simulink model "rotacao"  (R2016a)
settings: Solver=ode4  SolverMode=SingleTasking  StartTime=0.0  StopTime=80  FixedStep=0.001  RelTol=1e-3
undefined symbols (not defined in the file or in its folder): DiscIntNeverNeededParam, sigbuilder_block
settings Model: SimulationMode=accelerator  Creator=colom  LastModifiedBy=ITA
settings SolverCC: AutoInsertRateTranBlk=on
settings DataIOCC: ReturnWorkspaceOutputs=on
settings DebuggingCC: UnconnectedInputMsg=none  UnconnectedOutputMsg=none  UnconnectedLineMsg=none  SFUnexpectedBacktrackingDiag=error  SFNoUnconditionalDefaultTransitionDiag=error
settings HardwareCC: ProdWordSize=32  ProdHWDeviceType=Specified
settings SFSimCC: SimUseLocalCustomCode=on
settings RTWCC: RTWUseLocalCustomCode=on
settings GRTTargetCC: TargetLangStandard=C99 (ISO)  GeneratePreprocessorConditionals=Use local settings
settings ConfigComp: CovMetricSettings=dwe  CovHtmlReporting=off  CovSaveCumulativeToWorkspaceVar=off  CovSaveSingleToWorkspaceVar=off  CovExternalEMLEnable=on

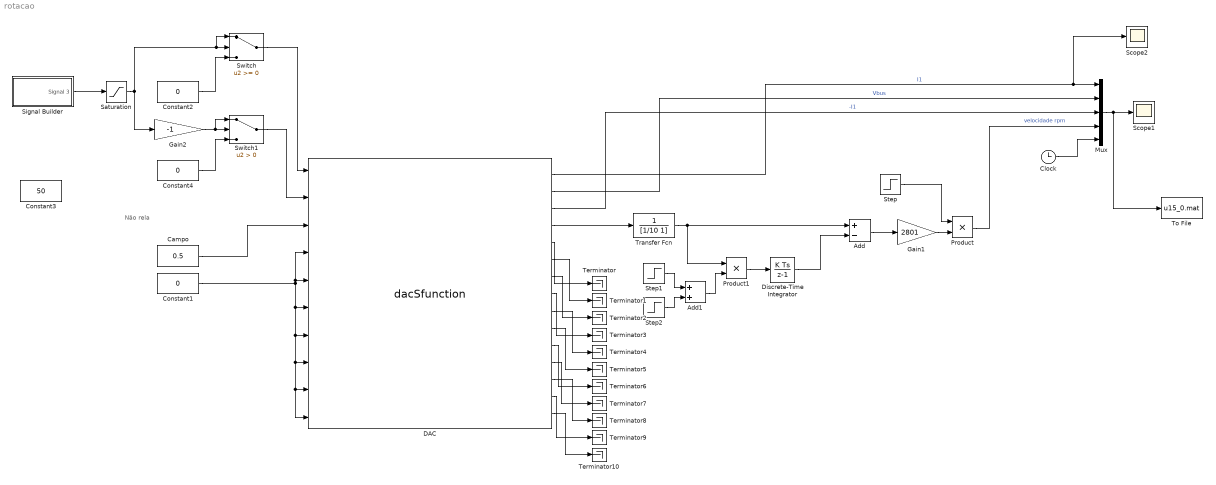
== system rotacao ==
  note: Não rela
  Add : Sum  Inputs=+-
  Add1 : Sum
  Campo : Constant  Value=0.5
  Clock : Clock
  Constant1 : Constant  Value=0
  Constant2 : Constant  Value=0
  Constant3 : Constant  Value=50
  Constant4 : Constant  Value=0
  DAC : S-Function  FunctionName=dacSfunction  Parameters=serialPort,sampleFreqHz,gpioCh1Mode,gpioCh1FinalState,gpioCh2Mode,gpioCh2FinalState,gpioCh3Mode,gpioCh3FinalState,gpioCh4Mode,gpioCh4FinalState,gpioCh5Mode,gpioCh5FinalState,gpioCh6Mode,gpioCh6FinalState,gpioCh7Mode,gpioCh7FinalState,pwmDeadTimeNs,pwmFrequencyHz,pwm1Mode,pwm1FastMode,pwm1ChPolarity,pwm1ChnPolarity,pwm1ChIdleState,pwm1ChnIdleState,pwm1FinalDuty,pwm2Mode,pwm2FastMode,pwm2ChPolarity,pwm2ChnPolarity,pwm2ChIdleState,pwm2ChnIdleState,pwm2FinalDuty,pwm3Mode,pwm3FastMode,pwm3ChPolarity,pwm3ChnPolarity,pwm3ChIdleState,pwm3ChnIdleState,pwm3FinalDuty,enc1Mode,enc1Quadrature,enc1Direction,enc1Filter,enc1ResetCount,enc2Mode,enc2Quadrature,enc2Direction,enc2Filter,enc2ResetCount,enc3Mode,enc3Quadrature,enc3Direction,enc3Filter,enc3ResetCount  SFunctionDeploymentMode=off  EnableBusSupport=off  mask{serialPort='COM4', sampleFreqHz=100, gpioCh1Mode=Input, gpioCh1FinalState=Low, gpioCh2Mode=Input, gpioCh2FinalState=Low, gpioCh3Mode=Output, gpioCh3FinalState=High, gpioCh4Mode=Input, gpioCh4FinalState=Low, gpioCh5Mode=Input, gpioCh5FinalState=Low, gpioCh6Mode=Input, gpioCh6FinalState=Low, gpioCh7Mode=Input, gpioCh7FinalState=Low, pwmFrequencyHz=20000, pwmDeadTimeNs=1000, pwm1Mode=Mode 1, pwm1FastMode=off, pwm1ChPolarity=HIGH, pwm1ChnPolarity=HIGH, pwm1ChIdleState=LOW, pwm1ChnIdleState=LOW, pwm1FinalDuty=0, pwm2Mode=Mode 1, pwm2FastMode=off, pwm2ChPolarity=HIGH, pwm2ChnPolarity=HIGH, pwm2ChIdleState=LOW, pwm2ChnIdleState=LOW, pwm2FinalDuty=0, pwm3Mode=Mode 1, pwm3FastMode=off, pwm3ChPolarity=HIGH, pwm3ChnPolarity=HIGH, pwm3ChIdleState=LOW, pwm3ChnIdleState=LOW, pwm3FinalDuty=0, enc1Mode=Counter, enc1Quadrature=High resolution, enc1Direction=Counter Clock Wise is positive, enc1Filter=15, enc1ResetCount=off, enc2Mode=Counter, enc2Quadrature=High resolution, enc2Direction=Counter Clock Wise is positive, enc2Filter=15, enc2ResetCount=off, enc3Mode=Counter, enc3Quadrature=High resolution, enc3Direction=Clock Wise is positive, enc3Filter=15, enc3ResetCount=off}
      mask prompts: serialPort "Serial port"; sampleFreqHz "Sample frequency (Hz)"; gpioCh1Mode "Mode"; gpioCh1FinalState "Final state"; gpioCh2Mode "Mode"; gpioCh2FinalState "Final state"; gpioCh3Mode "Mode"; gpioCh3FinalState "Final state"; gpioCh4Mode "Mode"; gpioCh4FinalState "Final state"; gpioCh5Mode "Mode"; gpioCh5FinalState "Final state"; gpioCh6Mode "Mode"; gpioCh6FinalState "Final state"; gpioCh7Mode "Mode"; gpioCh7FinalState "Final state"; pwmFrequencyHz "Frequency (Hz)"; pwmDeadTimeNs "Dead time (ns)"; pwm1Mode "Mode"; pwm1FastMode "Fast mode"; pwm1ChPolarity "CH polarity"; pwm1ChnPolarity "CHN polarity"; pwm1ChIdleState "CH idle state"; pwm1ChnIdleState "CHN idle state"; pwm1FinalDuty "Final duty"; pwm2Mode "Mode"; pwm2FastMode "Fast mode"; pwm2ChPolarity "CH polarity"; pwm2ChnPolarity "CHN polarity"; pwm2ChIdleState "CH idle state"; pwm2ChnIdleState "CHN idle state"; pwm2FinalDuty "Final duty"; pwm3Mode "Mode"; pwm3FastMode "Fast mode"; pwm3ChPolarity "CH polarity"; pwm3ChnPolarity "CHN polarity"; pwm3ChIdleState "CH idle state"; pwm3ChnIdleState "CHN idle state"; pwm3FinalDuty "Final duty"; enc1Mode "Mode"; enc1Quadrature "Resolution"; enc1Direction "Direction"; enc1Filter "Filter"; enc1ResetCount "Reset count"; enc2Mode "Mode"; enc2Quadrature "Resolution"; enc2Direction "Direction"; enc2Filter "Filter"; enc2ResetCount "Reset count"; enc3Mode "Mode"; enc3Quadrature "Resolution"; enc3Direction "Direction"; enc3Filter "Filter"; enc3ResetCount "Reset count"
      mask init:
      | % The first list item is initiated with 1 and not 0
      mask TypeOptions gpioCh1Mode: Input | Output
      mask TypeOptions gpioCh1FinalState: Low | High
      mask TypeOptions gpioCh2Mode: Input | Output
      mask TypeOptions gpioCh2FinalState: Low | High
      mask TypeOptions gpioCh3Mode: Input | Output
      mask TypeOptions gpioCh3FinalState: Low | High
      mask TypeOptions gpioCh4Mode: Input | Output
      mask TypeOptions gpioCh4FinalState: Low | High
      mask TypeOptions gpioCh5Mode: Input | Output
      mask TypeOptions gpioCh5FinalState: Low | High
      mask TypeOptions gpioCh6Mode: Input | Output
      mask TypeOptions gpioCh6FinalState: Low | High
      mask TypeOptions gpioCh7Mode: Input | Output
      mask TypeOptions gpioCh7FinalState: Low | High
      mask TypeOptions pwm1Mode: Mode 1 | Mode 2
      mask TypeOptions pwm1ChPolarity: LOW | HIGH
      mask TypeOptions pwm1ChnPolarity: LOW | HIGH
      mask TypeOptions pwm1ChIdleState: LOW | HIGH
      mask TypeOptions pwm1ChnIdleState: LOW | HIGH
      mask TypeOptions pwm2Mode: Mode 1 | Mode 2
      mask TypeOptions pwm2ChPolarity: LOW | HIGH
      mask TypeOptions pwm2ChnPolarity: LOW | HIGH
      mask TypeOptions pwm2ChIdleState: LOW | HIGH
      mask TypeOptions pwm2ChnIdleState: LOW | HIGH
      mask TypeOptions pwm3Mode: Mode 1 | Mode 2
      mask TypeOptions pwm3ChPolarity: LOW | HIGH
      mask TypeOptions pwm3ChnPolarity: LOW | HIGH
      mask TypeOptions pwm3ChIdleState: LOW | HIGH
      mask TypeOptions pwm3ChnIdleState: LOW | HIGH
      mask TypeOptions enc1Mode: Counter | Time measurement
      mask TypeOptions enc1Quadrature: Low resolution | High resolution
      mask TypeOptions enc1Direction: Counter Clock Wise is positive | Clock Wise is positive
      mask TypeOptions enc2Mode: Counter | Time measurement
      mask TypeOptions enc2Quadrature: Low resolution | High resolution
      mask TypeOptions enc2Direction: Counter Clock Wise is positive | Clock Wise is positive
      mask TypeOptions enc3Mode: Counter | Time measurement
      mask TypeOptions enc3Quadrature: Low resolution | High resolution
      mask TypeOptions enc3Direction: Counter Clock Wise is positive | Clock Wise is positive
      mask DialogControl DescTextVar Prompt: %<MaskDescription> OpenDAC configuration
      mask Display:
      | % Give names to the input ports
      | port_label('input',  1, 'PWM CH1 (PA8/PB13)');
      | port_label('input',  2, 'PWM CH2 (PA9/PB14)');
      | port_label('input',  3, 'PWM CH3 (PA10/PB15)');
      | port_label('input',  4, 'Digital Write CH1 (PC15)');
      | port_label('input',  5, 'Digital Write CH2 (PC14)');
      | port_label('input',  6, 'Digital Write CH3 (PC13)');
      | port_label('input',  7, 'Digital Write CH4 (PB9)');
      | port_label('input',  8, 'Digital Write CH5 (PB8)');
      | port_label('input',  9, 'Digital Write CH6 (PB1)');
      | port_label('input', 10, 'Digital Write CH7 (PB12)');
      | 
      | % Give names to the output ports
      | port_label('output',  1, 'Analog In CH1 (PA0)');
      | port_label('output',  2, 'Analog In CH2 (PA1)');
      | port_label('output',  3, 'Analog In CH3 (PA4)');
      | port_label('output',  4, 'Analog In CH4 (PB0)');
      | port_label('output',  5, 'Encoder 1 (PB6/PB7)');
      | port_label('output',  6, 'Encoder 2 (PA15/PB3)');
      | port_label('output',  7, 'Encoder 3 (PB4/PB5)');
      | port_label('output',  8, 'Digital Read CH1 (PC15)');
      | port_label('output',  9, 'Digital Read CH2 (PC14)');
      | port_label('output', 10, 'Digital Read CH3 (PC13)');
      | port_label('output', 11, 'Digital Read CH4 (PB9)');
      | port_label('output', 12, 'Digital Read CH5 (PB8)');
      | port_label('output', 13, 'Digital Read CH6 (PB1)');
      | port_label('output', 14, 'Digital Read CH7 (PB12)');
      | port_label('output', 15, 'Real Time Clock');
  Discrete-Time Integrator : DiscreteIntegrator  InitialConditionSetting=State (most efficient)  ICPrevOutput=DiscIntNeverNeededParam  ICPrevScaledInput=DiscIntNeverNeededParam
  Gain1 : Gain  Gain=2801
  Gain2 : Gain  Gain=-1
  Mux : Mux  Inputs=5
  Product : Product
  Product1 : Product
  Saturation : Saturate  UpperLimit=1  LowerLimit=-1
  Scope1 : Scope
  Scope2 : Scope
  Signal Builder : Subsystem  Tag=STV Subsys  LoadFcn=sigbuilder_block('load',[6 30 948 639.75 ]);  StartFcn=sigbuilder_block('start');  StopFcn=sigbuilder_block('stop');  ClipboardFcn=sigbuilder_block('clipboard');  mask(Sigbuilder block){}
      mask help: Simulink:masks:SigbuilderBlock_MD
      mask init:
      | if ~strcmp(get_param(bdroot(gcbh),'SimulationStatus'),'stopped') tuvar = sigbuilder_block('maskInit'); end
      settings: CopyFcn=sigbuilder_block('copy');  DeleteFcn=sigbuilder_block('delete');  ModelCloseFcn=sigbuilder_block('modelClose');  PreSaveFcn=sigbuilder_block('preSave');  PauseFcn=sigbuilder_block('pause');  ContinueFcn=sigbuilder_block('continue');  NameChangeFcn=sigbuilder_block('namechange');  OpenFcn=sigbuilder_block('open',[6 30 948 639.75 ]);  CloseFcn=sigbuilder_block('close');
      mask Display: plot(0, 0, 100, 100,[2, 2, 32, 32, 2], [68, 8, 8, 68, 68],[32, 2], [38, 38], [32, 19, 2],[53, 60, 44], [32, 17, 17, 2],[16, 16, 31, 31]);txt = getActiveGroup(gcbh);text(2, 100, txt,'verticalAlignment', 'top');
  Step : Step  Time=2  SampleTime=0
  Step1 : Step  Time=0.99  SampleTime=0
  Step2 : Step  Time=1.01  After=-1  SampleTime=0
  Switch : Switch
  Switch1 : Switch  Criteria=u2 > Threshold
  Terminator{,1..10} (11 alike) : Terminator
  To File : ToFile  Filename=u15_0.mat  MatrixName=data
  Transfer Fcn : TransferFcn  Denominator=[1/10 1]
  wires:
  Campo/1 -> DAC/3
  DAC/9 -> Terminator4/1
  DAC/5 -> Terminator/1
  DAC/14 -> Terminator9/1
  DAC/6 -> Terminator1/1
  DAC/8 -> Terminator3/1
  DAC/7 -> Terminator2/1
  DAC/13 -> Terminator8/1
  DAC/12 -> Terminator7/1
  DAC/2 -> Mux/2  "Vbus"
  DAC/1 -> Scope2/1, Mux/1  "I1"
  DAC/3 -> Mux/3  "-I1"
  DAC/15 -> Terminator10/1
  DAC/10 -> Terminator5/1
  DAC/11 -> Terminator6/1
  Constant1/1 -> DAC/4, DAC/5, DAC/8, DAC/9, DAC/10, DAC/7, DAC/6
  Mux/1 -> To File/1, Scope1/1
  Constant2/1 -> Switch/3
  Constant4/1 -> Switch1/3
  Gain2/1 -> Switch1/2, Switch1/1
  Saturation/1 -> Switch/1, Switch/2, Gain2/1
  Switch1/1 -> DAC/2
  Switch/1 -> DAC/1
  Add/1 -> Gain1/1
  Gain1/1 -> Product/2
  Step/1 -> Product/1
  Product/1 -> Mux/4  "velocidade rpm"
  Transfer Fcn/1 -> Product1/1, Add/1
  Step1/1 -> Add1/1
  Step2/1 -> Add1/2
  Add1/1 -> Product1/2
  Product1/1 -> Discrete-Time Integrator/1
  Discrete-Time Integrator/1 -> Add/2
  DAC/4 -> Transfer Fcn/1
  Clock/1 -> Mux/5
  Signal Builder/1(Signal 3) -> Saturation/1

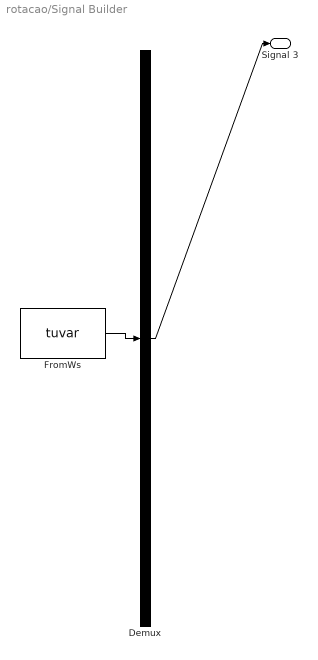
== system rotacao/Signal Builder ==
  Demux : Demux  Tag=STV Demux  Outputs=1
  FromWs : FromWorkspace  Tag=STV FromWs  VariableName=tuvar  SampleTime=0
      SigBuilderData=|
      | common.afterFinalStr = 'Extrapolate'
      | common.sampleTime = 0
      | dataSet.timeRange = [0 100]
      | dataSet.name = 'Group 1'
      | sbobj.Groups.Name = 'Group 1'
      | sbobj.Groups.Signals.Name = 'Signal 3'
      | sbobj.Groups.Signals.XData = [0 3 15 30 30 100]
      | sbobj.Groups.Signals.YData = [0 0 0.4 0.4 0.45 0.45]
      | sbobj.Groups.TimeRange = [0 100]
  Signal 3 : Outport  Tag=STV Outport
  wires:
  FromWs/1 -> Demux/1
  Demux/1 -> Signal 3/1
